simulink model "Keyboard_in2"  (R2020a)
settings: Solver=FixedStepDiscrete  StartTime=0.0  StopTime=Inf  RelTol=1e-3  EnableMultiTasking=on
libraries: robotlib x2
settings Model: Creator=pit  LastModifiedBy=grady
settings DataIOCC: LimitDataPoints=on  SaveFormat=Array  SignalLoggingSaveFormat=ModelDataLogs  ReturnWorkspaceOutputs=off
settings OptimizationCC: ExpressionDepthLimit=2147483647  InitFltsAndDblsToZero=on  LifeSpan=inf
settings DebuggingCC: UnderspecifiedInitializationDetection=Classic  MergeDetectMultiDrivingBlocksExec=none  SolverPrmCheckMsg=warning  FcnCallInpInsideContextMsg=warning  StateNameClashWarn=warning  SFUnexpectedBacktrackingDiag=warning  SFNoUnconditionalDefaultTransitionDiag=warning  SFExecutionAtInitializationDiag=none  ArithmeticOperatorsInVariantConditions=warning
settings HardwareCC: ProdBitPerPointer=32  ProdBitPerSizeT=32  ProdBitPerPtrDiffT=32  ProdLargestAtomicFloat=None  ProdIntDivRoundTo=Undefined  ProdEndianess=Unspecified  ProdWordSize=32  ProdHWDeviceType=32-bit Generic
settings ModelReferenceCC: PropagateSignalLabelsOutOfModel=off
settings SFSimCC: SimUseLocalCustomCode=off  CustomCodeUndefinedFunction=UseInterfaceOnly
settings RTWCC: RTWUseLocalCustomCode=off
settings CodeAppCC: StateflowObjectComments=on
settings GRTTargetCC: TargetLangStandard=C89/C90 (ANSI)  CombineOutputUpdateFcns=off  GRTInterface=on
settings ConfigComp: CovMetricSettings=dw  CovHtmlReporting=on  CovSaveCumulativeToWorkspaceVar=on  CovSaveSingleToWorkspaceVar=on  CovExternalEMLEnable=off  CovSFcnEnable=off

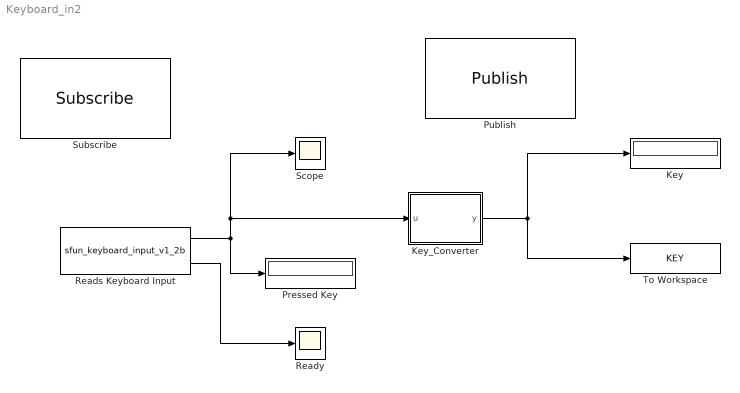
== system Keyboard_in2 ==
  Key : Display
  Key_Converter : MATLAB Function  TreatAsAtomicUnit=on
  Pressed Key : Display
  Publish : robotlib/Publish  topicSource=Specify your own  topic=/cmd_vel  messageType=rosgraph_msgs/Log  messageQueueLength=1
  Reads Keyboard Input : M-S-Function  FunctionName=sfun_keyboard_input_v1_2b  mask(Keyboard Input){}
      mask help: Keyboard Input
      mask Display: fprintf('Keyboard');
  Ready : Scope
  Scope : Scope
  Subscribe : robotlib/Subscribe  topicSource=Select from ROS network  topic=/my_topic  messageType=geometry_msgs/Point  sampleTime=-1  messageQueueLength=1
  To Workspace : ToWorkspace  VariableName=KEY  SampleTime=-1
      settings: Save2DSignal=2-D array (concatenate along first dimension)
  wires:
  Reads Keyboard Input/1 -> Scope/1, Key_Converter/1(u), Pressed Key/1
  Reads Keyboard Input/2 -> Ready/1
  Key_Converter/1(y) -> To Workspace/1, Key/1

== matlab function Keyboard_in2/Key_Converter ==
  data: u input; y output
function y = KeyConvert(u)

%key converter from ASCII to letter.
out=0;
if(u==119)
    %w
    out=1;
elseif(u==120)
    %x
    out=2;
elseif(u==97)
    %a
    out=3;
elseif(u==100)
    %d
    out=4;
elseif(u==115)
    %s
    out=5;
elseif(u==121)
    %TURN OFF ROS CONNECTION
end

y = out;
